simulink model "convert_1"  (R2021a)
settings: Solver=VariableStepAuto  StartTime=0.0  StopTime=10.0  RelTol=1e-3
settings Model: Creator=yasso  LastModifiedBy=yasso

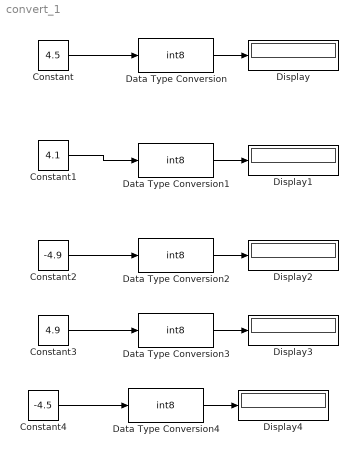
== system convert_1 ==
  Constant : Constant  Value=4.5
  Constant1 : Constant  Value=4.1
  Constant2 : Constant  Value=-4.9
  Constant3 : Constant  Value=4.9
  Constant4 : Constant  Value=-4.5
  Data Type Conversion : DataTypeConversion  OutDataTypeStr=int8  RndMeth=Round
  Data Type Conversion1 : DataTypeConversion  OutDataTypeStr=int8  RndMeth=Nearest
  Data Type Conversion2 : DataTypeConversion  OutDataTypeStr=int8  RndMeth=Nearest
  Data Type Conversion3 : DataTypeConversion  OutDataTypeStr=int8  RndMeth=Zero
  Data Type Conversion4 : DataTypeConversion  OutDataTypeStr=int8  RndMeth=Round
  Display{,1..4} (5 alike) : Display
  wires:
  Constant/1 -> Data Type Conversion/1
  Data Type Conversion/1 -> Display/1
  Constant1/1 -> Data Type Conversion1/1
  Data Type Conversion1/1 -> Display1/1
  Data Type Conversion2/1 -> Display2/1
  Constant2/1 -> Data Type Conversion2/1
  Constant3/1 -> Data Type Conversion3/1
  Data Type Conversion3/1 -> Display3/1
  Data Type Conversion4/1 -> Display4/1
  Constant4/1 -> Data Type Conversion4/1
